simulink library "vmc"  (R2021b)
settings: Solver=VariableStepAuto  StartTime=0.0  StopTime=10.0  RelTol=1e-3
undefined symbols (not defined in the file or in its folder): AVMC_ACCDeltaTqIGain_X_kph, AVMC_ACCDeltaTqIGain_Y_mps2, AVMC_ACCDeltaTqIGainP2_X_kph, AVMC_ACCDeltaTqIGainP2_Y_mps2, AVMC_ACCDeltaTqPGain_X_kph, AVMC_ACCDeltaTqPGain_Y_kph, AVMC_ACCDeltaTqPGainP2_X_kph, AVMC_ACCDeltaTqPGainP2_Y_kph, AVMC_ACCLongSteadyCtrl_X_kph, AVMC_CCAccelCMD_X_kph, AVMC_CCAccelCMD_Y_kph, AVMC_CCDeltaTqIGain_X_kph, AVMC_CCDeltaTqIGain_Y_mps2, AVMC_CCDeltaTqPGain_X_kph, AVMC_CCDeltaTqPGain_Y_kph, AVMC_CCLongSteadyCtrl_X_kph, AVMC_DISCDeltaTqIGainP2_X_kph, AVMC_DISCDeltaTqIGainP2_Y_mps2, AVMC_ESCRegenOut_X_kph, AVMC_ESCRegenOut_Y_Deg, AVMC_ESCRegenOutEnSpd_X_Deg, AVMC_LatESCRegenOut_X_kph, AVMC_LatESCRegenOut_Y_Deg, AVMC_LongAccDeadZone_X_kph, AVMC_LongAccDeadZoneP2_X_kph, AVMC_LongAccFiltTs_X_Gps, AVMC_LongAccFiltTsP2_X_Gps, AVMC_MCPresBaseTq_X_bar, AVMC_MSAAccelCMD_X_kph, AVMC_MSAAccelCMD_Y_kph, AVMC_MSADeltaTqIGain_X_kph, AVMC_MSADeltaTqIGain_Y_mps2, AVMC_MSADeltaTqPGain_X_kph, AVMC_MSADeltaTqPGain_Y_kph, AVMC_MSALongSteadyCtrl_X_kph, AVMC_MSAPedalOvrd_X_kph, AVMC_MSASpdBand_X_kph, AVMC_OPDDisSlideRate_X_Deg, AVMC_RDCDetectTime_X_kph, AVMC_RDCDetectTime_Y_pct, AVMC_RDCEnSlideRate_X_Deg, AVMC_StESCYaw_X_kph, AVMC_StESCYaw_Y_Deg, AVMC_StESCYawCom_X_kph, AVMC_StESCYawCom_Y_Gps, AVMC_TMSpdBaseTq_X_rpm, C_TASK_10MS_S, C_TASK_5MS_S, DEG2RAD, Discrete, ENUM_ADASACCSTA_ACTIVE, ENUM_ADASACCSTA_OVERRIDE, ENUM_ADASACCSTA_STANDBY, ENUM_ADASMSASTA_ACTIVE, ENUM_ADASMSASTA_ERROR, ENUM_ADASMSASTA_OFF, ENUM_ADASMSASTA_OVERSPEED, ENUM_ADASMSASTA_STANDBY, ENUM_ADASMSASTA_UNDERSPEED, ENUM_ADASMSASTA_UNLIMIT ... (+254)
libraries: hcu_lib x57, simulink x49, ctrlSharedLib x6, simulink_extras x1
(part 1 of 9)
settings Model: Creator=FVT22120  LastModifiedBy=FVT23010

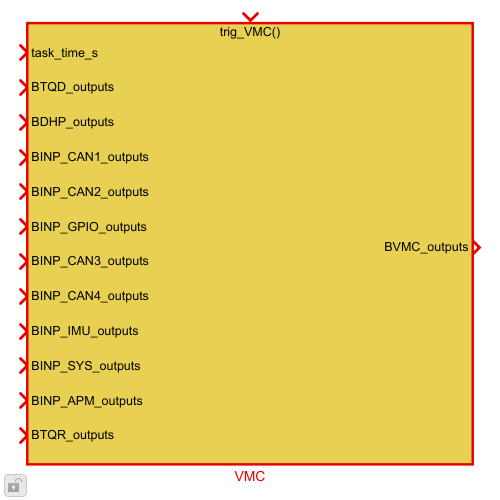
[thumbnail: Simulink's stored preview of the top-level diagram]
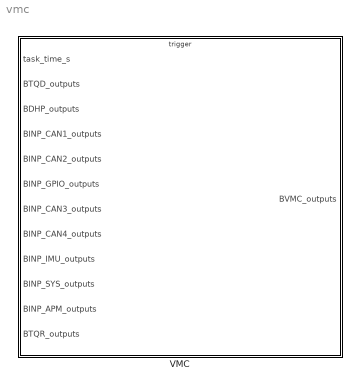
== system vmc ==
  VMC : Subsystem
      settings: RTWSystemCode=Nonreusable function  RTWFcnNameOpts=Use subsystem name  RTWFileNameOpts=Use subsystem name

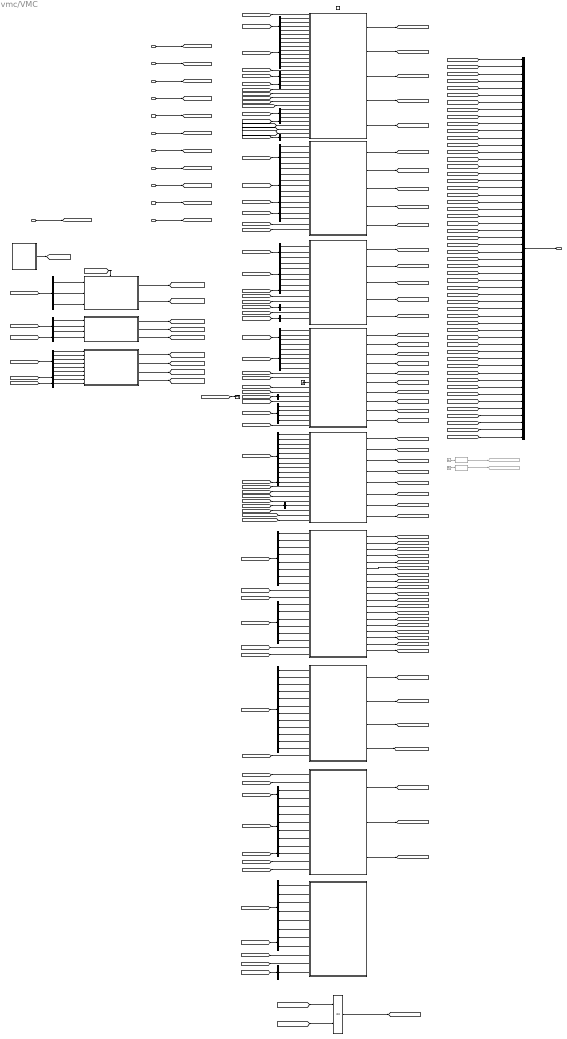
== system vmc/VMC ==
  note: Phase2_WAdd
  task_time_s : Inport
  BTQD_outputs : Inport  Port=2  OutDataTypeStr=Bus: BTQD_outputs
  BDHP_outputs : Inport  Port=3  OutDataTypeStr=Bus: BDHP_outputs
  BINP_CAN1_outputs : Inport  Port=4  OutDataTypeStr=Bus: BINP_CAN1_outputs
  BINP_CAN2_outputs : Inport  Port=5  OutDataTypeStr=Bus: BINP_CAN2_outputs  LockScale=on
  BINP_GPIO_outputs : Inport  Port=6  OutDataTypeStr=Bus: BINP_GPIO_outputs
  BINP_CAN3_outputs : Inport  Port=7  OutDataTypeStr=Bus: BINP_CAN3_outputs
  BINP_CAN4_outputs : Inport  Port=8  OutDataTypeStr=Bus: BINP_CAN4_outputs
  BINP_IMU_outputs : Inport  Port=9  OutDataTypeStr=Bus: BINP_IMU_outputs
  BINP_SYS_outputs : Inport  Port=10  OutDataTypeStr=Bus: BINP_SYS_outputs
  BINP_APM_outputs : Inport  Port=11  OutDataTypeStr=Bus: BINP_APM_outputs
  BTQR_outputs : Inport  Port=12  OutDataTypeStr=Bus: BTQR_outputs
  trig_VMC : TriggerPort  TriggerType=function-call  VariantControl=(inherit)  PortDimensions=1
  ACC_Function : Subsystem
  ACC_ReqAccelControl : Subsystem
  APS function : Subsystem
  Bus Creator : BusCreator  Inputs=54  OutDataTypeStr=Bus:BVMC_outputs  NonVirtualBus=on
  Bus Selector : BusSelector  OutputSignals=VINP_ACCRequiredAccel_mps2,VINP_ADASACCSta_enum,VINP_VehSpeed_kph,VINP_ACCSetSpeed_enum,VINP_ACCVehHoldReq_flg,VINP_MCPressure_bar,VINP_ESCADASSta_enum,VINP_TargetType_enum
  Bus Selector1 : BusSelector  OutputSignals=VTQD_ExternalTqAllow_flg,VTQD_DriverWhlTqDem_Nm,VTQD_LowIdleAccPedal_flg,VTQD_GearActualPosn_enum,VTQD_ExtDoorAllow_flg
  Bus Selector10 : BusSelector  OutputSignals=VINP_MemOffsetGyroX_raw16,VINP_MemOffsetGyroY_raw16,VINP_MemOffsetGyroZ_raw16,VINP_MemOffsetAccX_raw16,VINP_MemOffsetAccY_raw16,VINP_MemOffsetAccZ_raw16,VINP_SensingGyroX_raw16,VINP_SensingGyroY_raw16,VINP_SensingGyroZ_raw16,VINP_SensingAccX_raw16,VINP_SensingAccY_raw16,VINP_SensingAccZ_raw16
  Bus Selector11 : BusSelector  OutputSignals=VTQD_ExternalTqAllow_flg,VTQD_ExtShftAllow_flg,VTQD_ExtDoorAllow_flg,VTQD_GearActualPosn_enum
  Bus Selector12 : BusSelector  OutputSignals=VDHP_ActAPSPosn_pct
  Bus Selector13 : BusSelector  OutputSignals=VINP_GRADE_Deg,VINP_LatAccel_Gps,VINP_LongAccel_Gps,VINP_VehSpeed_kph,VINP_LFRawWhlSpeed_kph,VINP_RFRawWhlSpeed_kph,VINP_LRRawWhlSpeed_kph,VINP_RRRawWhlSpeed_kph,VINP_ACCSetSpeed_enum,VINP_TargetType_enum
  Bus Selector14 : BusSelector  OutputSignals=VINP_RegenMode_enum,VINP_SWCResUpSta_flg
  Bus Selector15 : BusSelector  OutputSignals=VINP_GPSLAT_s,VINP_GPSLONG_enum
  Bus Selector16 : BusSelector  OutputSignals=VINP_SetSpd_kph
  Bus Selector17 : BusSelector  OutputSignals=VINP_LFRawWhlSpeed_kph,VINP_RFRawWhlSpeed_kph,VINP_LRRawWhlSpeed_kph,VINP_RRRawWhlSpeed_kph,VINP_VehSpeed_kph,VINP_BrkPedalPos_pct,VINP_BrkSwSta_flg,VINP_LongAccel_Gps
  Bus Selector18 : BusSelector  OutputSignals=VTQD_AfterAvailableTqDemFr_Nm,VTQD_AfterAvailableTqDemRr_Nm,VTQD_EquivAccPedalSWSta_flg,VTQD_GearActualPosn_enum,VTQD_RegenMode_enum,VTQD_VehActSpd_kph
  Bus Selector19 : BusSelector  OutputSignals=VTQD_AfterAvailableTqDemFr_Nm,VTQD_AfterAvailableTqDemRr_Nm
  Bus Selector2 : BusSelector  OutputSignals=VTQD_DriverWhlTqDem_Nm,VTQD_ExternalTqAllow_flg,VTQD_LowIdleAccPedal_flg,VTQD_ExtDoorAllow_flg,VTQD_CreepBaseTqD_Nm
  Bus Selector20 : BusSelector  OutputSignals=VINP_ESCActive_flg,VINP_SASAngle_Deg,VINP_LatAccel_Gps,VINP_VehSpeed_kph,VINP_YawRate_degps,VINP_RDCActive_enum
  Bus Selector21 : BusSelector  OutputSignals=VINP_HoodSW_flg
  Bus Selector22 : BusSelector  OutputSignals=VINP_LFRawWhlSpeed_kph,VINP_RFRawWhlSpeed_kph,VINP_LRRawWhlSpeed_kph,VINP_RRRawWhlSpeed_kph,VINP_VehSpeed_kph,VINP_LongAccel_Gps
  Bus Selector23 : BusSelector  OutputSignals=VTQD_GearActualPosn_enum
  Bus Selector24 : BusSelector  OutputSignals=VINP_DIDGetDynoMode_flg
  Bus Selector25 : BusSelector  OutputSignals=VINP_DIDGetDynoMode_flg
  Bus Selector26 : BusSelector  OutputSignals=VINP_APSStaSystem_enum,VINP_APSVMCReqA_flg,VINP_APSShiftPosnReq_enum,VINP_APSSpeedCMD_kph,VINP_CAASVMCReqA_flg
  Bus Selector27 : BusSelector  OutputSignals=VINP_VehSpeed_kph
  Bus Selector28 : BusSelector  OutputSignals=VINP_VehSpeed_kph,VINP_ACCRequiredAccel_mps2,VINP_ADASACCSta_enum
  Bus Selector29 : BusSelector  OutputSignals=VINP_METERKPHCalcu_kph
  Bus Selector3 : BusSelector  OutputSignals=VINP_BrkSwSta_flg,VINP_VehSpeed_kph,VINP_BrkPedalPos_pct
  Bus Selector30 : BusSelector  OutputSignals=VINP_VehSpeed_kph,VINP_ACCRequiredAccel_mps2,VINP_ACCVehHoldReq_flg,VINP_ACCObjRelSpd_mps,VINP_ACCObjDist_m,VINP_TimeGapLevel_enum
  Bus Selector31 : BusSelector  OutputSignals=VTQD_FrEDUAvailBrkRgnTq_Nm,VTQD_RrEDUAvailBrkRgnTq_Nm
  Bus Selector32 : BusSelector  OutputSignals=VINP_VehSpeed_kph,VINP_LongAccel_Gps,VINP_GRADE_Deg
  Bus Selector33 : BusSelector  OutputSignals=VTQR_FrTMTqReq_Nm,VTQR_RrTMTqReq_Nm,VTQR_ACCHoldPdovrdInc_flg
  Bus Selector34 : BusSelector  OutputSignals=VINP_FrTMSpd_rpm,VINP_RrTMSpd_rpm
  Bus Selector35 : BusSelector  OutputSignals=VINP_METERKPHCalcu_kph
  Bus Selector36 : BusSelector  OutputSignals=VINP_METERKPHCalcu_kph
  Bus Selector37 : BusSelector  OutputSignals=VINP_ADASACCSta_enum,VINP_MCPressure_bar,VINP_BrkSwSta_flg,VINP_BrkPedalPos_pct
  Bus Selector4 : BusSelector  OutputSignals=VDHP_ActAPSPosn_pct
  Bus Selector5 : BusSelector  OutputSignals=VTQD_ExternalTqAllow_flg,VTQD_DriverWhlTqDem_Nm,VTQD_GearActualPosn_enum
  Bus Selector6 : BusSelector  OutputSignals=VINP_VehSpeed_kph
  Bus Selector7 : BusSelector  OutputSignals=VINP_ZoneSpdCtrlMode_enum,VINP_SetSpd_kph,VINP_SWCCANCELSta_flg,VINP_SWCResUpSta_flg,VINP_SWCSetdownSta_flg
  Bus Selector8 : BusSelector  OutputSignals=VINP_BrakeSWGPIO_flg
  Bus Selector9 : BusSelector  OutputSignals=VINP_ZoneSpdCtrlMode_enum,VINP_SetSpd_kph,VINP_SWCResUpSta_flg,VINP_SWCSetdownSta_flg,VINP_SWCCANCELSta_flg
  CruiseControlFunction : Subsystem
  Data Type Conversion : DataTypeConversion  Commented=on  OutDataTypeStr=boolean
  Data Type Conversion1 : DataTypeConversion  Commented=on  OutDataTypeStr=boolean
  Goto62 : Goto  Commented=on  GotoTag=VVMC_CAASCtrlAvail_flg
  Goto63 : Goto  Commented=on  GotoTag=VVMC_CAASActive_flg
  Ground5 : Ground
  Ground7 : Ground  Commented=on
  Ground8 : Ground  Commented=on
  IMU : Subsystem
  Logical Operator : Logic  Operator=OR  AllPortsSameDT=off  OutDataTypeStr=boolean
  Long Acceleration Calculation : Subsystem
  LongAccel_EstSlope : Subsystem  TreatAsAtomicUnit=on
  MSA function : Subsystem
  RDC Determination : Subsystem
  Scheduler : Stateflow chart  TreatAsAtomicUnit=on
  Slide Rate  Calculation : Subsystem
  Subsystem1 : Subsystem
  Terminator1 : Terminator
  Vehicle Speed Estimation : Subsystem
  BVMC_outputs : Outport  OutDataTypeStr=Bus:BVMC_outputs
  wires:
  Bus Creator/1 -> BVMC_outputs/1  "BVMC_outputs"
  [VVMC_MSAWhlTqReq_Nm] -> Bus Creator/9
  [VVMC_ACCCtrlAvail_flg] -> Bus Creator/1
  [VVMC_CCPedalOvrd_flg] -> Bus Creator/16
  [VVMC_ADASWhlTqReq_Nm] -> Bus Creator/3
  [VVMC_ACCPedalOvrd_flg] -> Bus Creator/2
  [VVMC_MSAActive_flg] -> Bus Creator/11
  [VVMC_APSSpeedCMD_kph] -> Bus Creator/14
  [VVMC_MSACtrlSta_enum] -> Bus Creator/7
  [VVMC_APSCtrlAvail_flg] -> Bus Creator/12
  [VVMC_CruzActive_flg] -> Bus Creator/10
  [VVMC_APSActive_flg] -> Bus Creator/13
  [VVMC_ADASActive_flg] -> Bus Creator/4
  [VVMC_CCCtrlSta_enum] -> Bus Creator/5
  [VVMC_APSShiftPosnReq_enum] -> Bus Creator/15
  [VVMC_CruzWhlTqReq_Nm] -> Bus Creator/8
  [VVMC_CCMSASpdWar_flg] -> Bus Creator/6
  MSA function/4(VVMC_MSAActive_flg) -> [VVMC_MSAActive_flg]
  MSA function/3(VVMC_MSASpdWar_flg) -> [VVMC_MSASpdWar_flg]
  MSA function/2(VVMC_MSAWhlTqReq_Nm) -> [VVMC_MSAWhlTqReq_Nm]
  MSA function/1(VVMC_MSACtrlSta_enum) -> [VVMC_MSACtrlSta_enum]
  [VVMC_LongAcc_Gps] -> MSA function/10(VVMC_LongAcc_Gps)
  [BINP_CAN1_outputs] -> Bus Selector6/1
  Bus Selector7/2 -> MSA function/5(VINP_SetSpd_kph)  "<VINP_SetSpd_kph>"
  Bus Selector7/1 -> MSA function/4(VINP_ZoneSpdCrlMode_enum)  "<VINP_ZoneSpdCtrlMode_enum>"
  Bus Selector5/2 -> MSA function/2(VTQD_DriverWhlTqDem_Nm)  "<VTQD_DriverWhlTqDem_Nm>"
  Bus Selector5/1 -> MSA function/1(VTQD_ExternalTqAllow_flg)  "<VTQD_ExternalTqAllow_flg>"
  CruiseControlFunction/1(VVMC_CCCtrlSta_enum) -> [VVMC_CCCtrlSta_enum]
  CruiseControlFunction/3(VVMC_CruzWhlTqReq_N m) -> [VVMC_CruzWhlTqReq_Nm]
  CruiseControlFunction/5(VVMC_CCPedalOvrd_flg) -> [VVMC_CCPedalOvrd_flg]
  CruiseControlFunction/2(VVMC_CCSpdWar_flg) -> [VVMC_CCSpdWar_flg]
  CruiseControlFunction/4(VVMC_CruzActive_flg) -> [VVMC_CruzActive_flg]
  [VVMC_LongAcc_Gps] -> CruiseControlFunction/15(VVMC_LongAcc_Gps)
  Bus Selector3/2 -> CruiseControlFunction/13(VINP_VehSpeed_kph)  "<VINP_VehSpeed_kph>"
  Bus Selector3/1 -> CruiseControlFunction/12(VINP_BrkSwSta_flg)  "<VINP_BrkSwSta_flg>"
  Bus Selector8/1 -> CruiseControlFunction/11(VINP_BrakeSWGPIO_flg)  "<VINP_BrakeSWGPIO_flg>"
  Bus Selector9/5 -> CruiseControlFunction/10(VINP_SWCCANCELSta_flg)  "<VINP_SWCCANCELSta_flg>"
  Bus Selector9/4 -> CruiseControlFunction/9(VINP_SWCSetdownSta_flg)  "<VINP_SWCSetdownSta_flg>"
  Bus Selector9/3 -> CruiseControlFunction/8(VINP_SWCResUpSta_flg)  "<VINP_SWCResUpSta_flg>"
  Bus Selector9/2 -> CruiseControlFunction/7(VINP_SetSpd_kph)  "<VINP_SetSpd_kph>"
  Bus Selector9/1 -> CruiseControlFunction/6(VINP_ZoneSpdCrlMode_enum)  "<VINP_ZoneSpdCtrlMode_enum>"
  Bus Selector1/3 -> CruiseControlFunction/3(VTQD_LowIdleAccPedal_flg)  "<VTQD_LowIdleAccPedal_flg>"
  Bus Selector1/2 -> CruiseControlFunction/2(VTQD_DriverWhlTqDem_Nm)  "<VTQD_DriverWhlTqDem_Nm>"
  Bus Selector1/1 -> CruiseControlFunction/1(VTQD_ExternalTqAllow_flg)  "<VTQD_ExternalTqAllow_flg>"
  BINP_CAN2_outputs/1 -> [BINP_CAN2_outputs]
  task_time_s/1 -> [task_time_s]  "task_time_s"
  BTQD_outputs/1 -> [BTQD_outputs]
  [BTQD_outputs] -> Bus Selector1/1
  [BINP_CAN1_outputs] -> Bus Selector3/1
  [VVMC_CCSpdWar_flg] -> Logical Operator/1
  [VVMC_MSASpdWar_flg] -> Logical Operator/2
  Logical Operator/1 -> [VVMC_CCMSASpdWar_flg]  "VVMC_CCMSASpdWar_flg"
  [BTQD_outputs] -> Bus Selector5/1
  BINP_GPIO_outputs/1 -> [BINP_GPIO_outputs]
  [BINP_GPIO_outputs] -> Bus Selector8/1
  BINP_CAN3_outputs/1 -> [BINP_CAN3_outputs]
  [BINP_CAN4_outputs] -> Bus Selector7/1
  [BINP_CAN4_outputs] -> Bus Selector9/1
  BDHP_outputs/1 -> [BDHP_outputs]
  BINP_CAN1_outputs/1 -> [BINP_CAN1_outputs]
  [BTQD_outputs] -> Bus Selector11/1
  APS function/1(VVMC_APSCtrlAvail_flg) -> [VVMC_APSCtrlAvail_flg]
  APS function/4(VVMC_APSShiftPosnReq_enum) -> [VVMC_APSShiftPosnReq_enum]
  Long Acceleration Calculation/1(VVMC_LongAcc_Gps) -> [VVMC_LongAcc_Gps]
  APS function/3(VVMC_APSSpeedCMD_kph) -> [VVMC_APSSpeedCMD_kph]
  Bus Selector11/1 -> APS function/1(VTQD_ExternalTqAllow_flg)  "<VTQD_ExternalTqAllow_flg>"
  [task_time_s] -> APS function/10(task_time_s)  "task_time_s"
  APS function/2(VVMC_APSActive_flg) -> [VVMC_APSActive_flg]
  BINP_CAN4_outputs/1 -> [BINP_CAN4_outputs]
  [VVMC_LongAcc_Gps] -> Bus Creator/17
  [task_time_s] -> Long Acceleration Calculation/14(task_time_s)  "task_time_s"
  Bus Selector1/4 -> CruiseControlFunction/4(VTQD_GearActualPosn_enum)  "<VTQD_GearActualPosn_enum>"
  Bus Selector11/2 -> APS function/2(VTQD_ExtShiftAllow_flg)  "<VTQD_ExtShftAllow_flg>"
  [VVMC_ADASNegReq_flg] -> Bus Creator/18
  Bus Selector3/3 -> CruiseControlFunction/14(VINP_BrkPedalPos_pct)  "<VINP_BrkPedalPos_pct>"
  Bus Selector17/6 -> Slide Rate  Calculation/6(VINP_BrkPedalPos_pct)  "<VINP_BrkPedalPos_pct>"
  Bus Selector17/7 -> Slide Rate  Calculation/7(VINP_BrkSwSta_flg)  "<VINP_BrkSwSta_flg>"
  Bus Selector17/4 -> Slide Rate  Calculation/4(VINP_RRRawWhlSpeed_kph)  "<VINP_RRRawWhlSpeed_kph>"
  Slide Rate  Calculation/4(VVMC_LRWhlSpdSlideRate_pct) -> [VVMC_LRWhlSpdSlideRate_pct]
  Slide Rate  Calculation/14(VVMC_ActRFSlideRate_pct) -> [VVMC_ActRFSlideRate_pct]
  Slide Rate  Calculation/8(VVMC_LR4WhlSpdSlideRate_pct) -> [VVMC_LR4WhlSpdSlideRate_pct]
  Slide Rate  Calculation/15(VVMC_ActLRSlideRate_pct) -> [VVMC_ActLRSlideRate_pct]
  Slide Rate  Calculation/16(VVMC_ActRRSlideRate_pct) -> [VVMC_ActRRSlideRate_pct]
  Slide Rate  Calculation/1(VVMC_RawWhlSpdSlideRate_pct) -> [VVMC_RawWhlSpdSlideRate_pct]
  Slide Rate  Calculation/12(VVMC_ActMaxSlideRate_pct) -> [VVMC_ActMaxSlideRate_pct]
  Slide Rate  Calculation/3(VVMC_RFWhlSpdSlideRate_pct) -> [VVMC_RFWhlSpdSlideRate_pct]
  Slide Rate  Calculation/2(VVMC_LFWhlSpdSlideRate_pct) -> [VVMC_LFWhlSpdSlideRate_pct]
  Slide Rate  Calculation/9(VVMC_RR4WhlSpdSlideRate_pct) -> [VVMC_RR4WhlSpdSlideRate_pct]
  Slide Rate  Calculation/5(VVMC_RRWhlSpdSlideRate_pct) -> [VVMC_RRWhlSpdSlideRate_pct]
  Bus Selector18/3 -> Slide Rate  Calculation/13(VTQD_EquivAccPedalSWSta_flg)  "<VTQD_EquivAccPedalSWSta_flg>"
  Bus Selector18/1 -> Slide Rate  Calculation/11(VTQD_AfterAvailableTqDemFr_Nm)  "<VTQD_AfterAvailableTqDemFr_Nm>"
  Bus Selector17/2 -> Slide Rate  Calculation/2(VINP_RFRawWhlSpeed_kph)  "<VINP_RFRawWhlSpeed_kph>"
  Bus Selector17/5 -> Slide Rate  Calculation/5(VINP_VehSpeed_kph)  "<VINP_VehSpeed_kph>"
  Bus Selector17/3 -> Slide Rate  Calculation/3(VINP_LRRawWhlSpeed_kph)  "<VINP_LRRawWhlSpeed_kph>"
  [task_time_s] -> Slide Rate  Calculation/10(task_time_s)  "task_time_s"
  [BTQD_outputs] -> Bus Selector18/1
  [BINP_CAN1_outputs] -> Bus Selector17/1
  Slide Rate  Calculation/10(VVMC_PredictVehSpd_kph) -> [VVMC_PredictVehSpd_kph]
  [VVMC_LongAcc_Gps] -> Slide Rate  Calculation/9(VVMC_LongAcc_Gps)
  Slide Rate  Calculation/18(VVMC_AltRWhlSlideRate_pct) -> [VVMC_AltRWhlSlideRate_pct]
  Slide Rate  Calculation/17(VVMC_AltLWhlSlideRate_pct) -> [VVMC_AltLWhlSlideRate_pct]
  Bus Selector17/1 -> Slide Rate  Calculation/1(VINP_LFRawWhlSpeed_kph)  "<VINP_LFRawWhlSpeed_kph>"
  Slide Rate  Calculation/6(VVMC_LF4WhlSpdSlideRate_pct) -> [VVMC_LF4WhlSpdSlideRate_pct]
  Slide Rate  Calculation/7(VVMC_RF4WhlSpdSlideRate_pct) -> [VVMC_RF4WhlSpdSlideRate_pct]
  Slide Rate  Calculation/19(VVMC_AltWhlSlideRate_pct) -> [VVMC_AltWhlSlideRate_pct]
  Slide Rate  Calculation/13(VVMC_ActLFSlideRate_pct) -> [VVMC_ActLFSlideRate_pct]
  Bus Selector18/2 -> Slide Rate  Calculation/12(VTQD_AfterAvailableTqDemRr_Nm)  "<VTQD_AfterAvailableTqDemRr_Nm>"
  [VVMC_ADASActive_flg] -> Long Acceleration Calculation/12(VVMC_ADASActive_flg)
  Bus Selector16/1 -> Long Acceleration Calculation/11(VINP_SetSpd_kph)  "<VINP_SetSpd_kph>"
  Bus Selector13/9 -> Long Acceleration Calculation/9(VINP_ACCSetSpeed_enum)  "<VINP_ACCSetSpeed_enum>"
  Bus Selector13/7 -> Long Acceleration Calculation/7(VINP_LRRawWhlSpeed_kph)  "<VINP_LRRawWhlSpeed_kph>"
  Bus Selector13/6 -> Long Acceleration Calculation/6(VINP_RFRawWhlSpeed_kph)  "<VINP_RFRawWhlSpeed_kph>"
  Bus Selector13/5 -> Long Acceleration Calculation/5(VINP_LFRawWhlSpeed_kph)  "<VINP_LFRawWhlSpeed_kph>"
  Bus Selector13/4 -> Long Acceleration Calculation/4(VINP_VehSpeed_kph)  "<VINP_VehSpeed_kph>"
  Bus Selector13/3 -> Long Acceleration Calculation/3(VINP_LongAccel_Gps)  "<VINP_LongAccel_Gps>"
  [VVMC_CruzActive_flg] -> Long Acceleration Calculation/13(VVMC_CruzActive_flg)
  [BINP_CAN4_outputs] -> Bus Selector16/1
  Bus Selector13/2 -> Long Acceleration Calculation/2(VINP_LatAccel_Gps)  "<VINP_LatAccel_Gps>"
  Bus Selector13/1 -> Long Acceleration Calculation/1(VINP_GRADE_deg)  "<VINP_GRADE_Deg>"
  Bus Selector13/8 -> Long Acceleration Calculation/8(VINP_RRRawWhlSpeed_kph)  "<VINP_RRRawWhlSpeed_kph>"
  [BINP_CAN1_outputs] -> Bus Selector13/1
  Bus Selector13/10 -> Long Acceleration Calculation/10(VINP_TargetType_enum)  "<VINP_TargetType_enum>"
  Long Acceleration Calculation/2(VVMC_LFWhlSpeedRollAve_kph) -> [VVMC_LFWhlSpeedRollAve_kph]
  Long Acceleration Calculation/3(VVMC_RFWhlSpeedRollAve_kph) -> [VVMC_RFWhlSpeedRollAve_kph]
  Long Acceleration Calculation/4(VVMC_LRWhlSpeedRollAve_kph) -> [VVMC_LRWhlSpeedRollAve_kph]
  Long Acceleration Calculation/5(VVMC_RRWhlSpeedRollAve_kph) -> [VVMC_RRWhlSpeedRollAve_kph]
  Long Acceleration Calculation/6(VVMC_CalMeterSpeed_kph) -> [VVMC_CalMeterSpeed_kph]
  [BTQD_outputs] -> APS function/11(BTQD_outputs)  "BTQD_outputs"
  [VVMC_ADASActive_flg] -> APS function/13(VVMC_ADASActive_flg)
  APS function/5(VVMC_APSStaSys_enum) -> [VVMC_APSStaSys_enum]
  APS function/6(VVMC_APSDecReqA_flg) -> [VVMC_APSDecReqA_flg]
  APS function/7(VVMC_APSDecReq_mps2) -> [VVMC_APSDecReq_mps2]
  APS function/8(VVMC_APSReq_enum) -> [VVMC_APSReq_enum]
  Bus Selector5/3 -> MSA function/3(VTQD_GearActualPosn_enum)  "<VTQD_GearActualPosn_enum>"
  Bus Selector7/3 -> MSA function/6(VINP_SWCCANCELSta_flg)  "<VINP_SWCCANCELSta_flg>"
  Bus Selector6/1 -> MSA function/9(VINP_VehSpeed_kph)  "<VINP_VehSpeed_kph>"
  [BDHP_outputs] -> Bus Selector12/1
  [task_time_s] -> MSA function/11(task_time_s)  "task_time_s"
  Bus Selector12/1 -> MSA function/12(VDHP_ActAPSPosn_pct)  "<VDHP_ActAPSPosn_pct>"
  [VVMC_CalMeterSpeed_kph] -> MSA function/13(VVMC_CalMeterSpeed_kph)
  [VVMC_CalMeterSpeed_kph] -> CruiseControlFunction/16(VVMC_CalMeterSpeed_kph)
  [VVMC_APSStaSys_enum] -> Bus Creator/19
  [VVMC_APSDecReqA_flg] -> Bus Creator/20
  [VVMC_APSDecReq_mps2] -> Bus Creator/21
  [VVMC_APSReq_enum] -> Bus Creator/22
  [VVMC_LFWhlSpeedRollAve_kph] -> Bus Creator/23
  [VVMC_RFWhlSpeedRollAve_kph] -> Bus Creator/24
  [VVMC_LRWhlSpeedRollAve_kph] -> Bus Creator/25
  [VVMC_RRWhlSpeedRollAve_kph] -> Bus Creator/26
  [VVMC_RawWhlSpdSlideRate_pct] -> Bus Creator/27
  [VVMC_LFWhlSpdSlideRate_pct] -> Bus Creator/28
  [VVMC_RFWhlSpdSlideRate_pct] -> Bus Creator/29
  [VVMC_LRWhlSpdSlideRate_pct] -> Bus Creator/30
  [VVMC_RRWhlSpdSlideRate_pct] -> Bus Creator/31
  [VVMC_PredictVehSpd_kph] -> Bus Creator/32
  [VVMC_4WhlSpdSlideRate_pct] -> Bus Creator/33
  [VVMC_LF4WhlSpdSlideRate_pct] -> Bus Creator/34
  [VVMC_RF4WhlSpdSlideRate_pct] -> Bus Creator/35
  [VVMC_LR4WhlSpdSlideRate_pct] -> Bus Creator/36
  [VVMC_RR4WhlSpdSlideRate_pct] -> Bus Creator/37
  [VVMC_ActMaxSlideRate_pct] -> Bus Creator/38
  [VVMC_ActLFSlideRate_pct] -> Bus Creator/39
  [VVMC_ActRFSlideRate_pct] -> Bus Creator/40
  [VVMC_ActLRSlideRate_pct] -> Bus Creator/41
  [VVMC_ActRRSlideRate_pct] -> Bus Creator/42
  [VVMC_AltLWhlSlideRate_pct] -> Bus Creator/43
  [VVMC_AltRWhlSlideRate_pct] -> Bus Creator/44
  [VVMC_AltWhlSlideRate_pct] -> Bus Creator/45
  Bus Selector7/4 -> MSA function/7(VINP_SWCResUpSta_flg)  "<VINP_SWCResUpSta_flg>"
  Bus Selector7/5 -> MSA function/8(VINP_SWCSetdownSta_flg)  "<VINP_SWCSetdownSta_flg>"
  [VVMC_MSAActive_flg] -> Long Acceleration Calculation/15(VVMC_MSAActive_flg)
  Long Acceleration Calculation/7(VVMC_EstSlope_Deg) -> [VVMC_EstSlope_Deg]
  [VVMC_EstSlope_Deg] -> Bus Creator/46
  Slide Rate  Calculation/11(VVMC_4WhlSpdSlideRate_pct) -> [VVMC_4WhlSpdSlideRate_pct]
  Bus Selector21/1 -> MSA function/14(VINP_HoodSW_flg)  "<VINP_HoodSW_flg>"
  [BINP_GPIO_outputs] -> Bus Selector21/1
  [VVMC_RWDRDCActive_enum] -> Bus Creator/47
  Bus Selector1/5 -> CruiseControlFunction/5(VTQD_ExtDoorAllow_flg)  "<VTQD_ExtDoorAllow_flg>"
  Bus Selector11/3 -> APS function/3(VTQD_ExtDoorAllow_flg)  "<VTQD_ExtDoorAllow_flg>"
  BINP_IMU_outputs/1 -> [BINP_IMU_outputs]
  [BINP_IMU_outputs] -> Bus Selector10/1
  Bus Selector10/1 -> IMU/1(VINP_MemOffsetGyroX_raw16)  "<VINP_MemOffsetGyroX_raw16>"
  Bus Selector10/2 -> IMU/2(VINP_MemOffsetGyroY_raw16)  "<VINP_MemOffsetGyroY_raw16>"
  Bus Selector10/3 -> IMU/3(VINP_MemOffsetGyroZ_raw16)  "<VINP_MemOffsetGyroZ_raw16>"
  Bus Selector10/4 -> IMU/4(VINP_MemOffsetAccX_raw16)  "<VINP_MemOffsetAccX_raw16>"
  Bus Selector10/5 -> IMU/5(VINP_MemOffsetAccY_raw16)  "<VINP_MemOffsetAccY_raw16>"
  Bus Selector10/6 -> IMU/6(VINP_MemOffsetAccZ_raw16)  "<VINP_MemOffsetAccZ_raw16>"
  Bus Selector10/7 -> IMU/7(VINP_SensingGyroX_raw16)  "<VINP_SensingGyroX_raw16>"
  Bus Selector10/8 -> IMU/8(VINP_SensingGyroY_raw16)  "<VINP_SensingGyroY_raw16>"
  Bus Selector10/9 -> IMU/9(VINP_SensingGyroZ_raw16)  "<VINP_SensingGyroZ_raw16>"
  Bus Selector10/10 -> IMU/10(VINP_SensingAccX_raw16)  "<VINP_SensingAccX_raw16>"
  Bus Selector10/11 -> IMU/11(VINP_SensingAccY_raw16)  "<VINP_SensingAccY_raw16>"
  Bus Selector10/12 -> IMU/12(VINP_SensingAccZ_raw16)  "<VINP_SensingAccZ_raw16>"
  IMU/1(VVMC_IMUEnaCmd_flg) -> [VVMC_IMUEnaCmd_flg]
  [VVMC_IMUEnaCmd_flg] -> Bus Creator/48
  Bus Selector18/4 -> Slide Rate  Calculation/14(VTQD_GearActualPosn_enum)  "<VTQD_GearActualPosn_enum>"
  [BINP_CAN1_outputs] -> Bus Selector20/1
  Bus Selector20/4 -> RDC Determination/8(VINP_VehSpeed_kph)  "<VINP_VehSpeed_kph>"
  [VVMC_ActMaxSlideRate_pct] -> RDC Determination/2(VVMC_ActMaxSlideRate_pct)
  Bus Selector20/2 -> RDC Determination/6(VINP_SASAngle_Deg)  "<VINP_SASAngle_Deg>"
  Bus Selector19/1 -> RDC Determination/3(VTQD_AfterAvailableTqDemFr_Nm)  "<VTQD_AfterAvailableTqDemFr_Nm>"
  RDC Determination/1(VVMC_RWDRDCActive_enum) -> [VVMC_RWDRDCActive_enum]
  Bus Selector20/3 -> RDC Determination/7(VINP_LatAccel_Gps)  "<VINP_LatAccel_Gps>"
  [BTQD_outputs] -> Bus Selector19/1
  Bus Selector20/6 -> RDC Determination/10(VINP_RDCActive_enum)  "<VINP_RDCActive_enum>"
  Bus Selector20/5 -> RDC Determination/9(VINP_YawRate_degps)  "<VINP_YawRate_degps>"
  [task_time_s] -> RDC Determination/1(task_time_s)  "task_time_s"
  Bus Selector19/2 -> RDC Determination/4(VTQD_AfterAvailableTqDemRr_Nm)  "<VTQD_AfterAvailableTqDemRr_Nm>"
  Bus Selector20/1 -> RDC Determination/5(VINP_ESCActive_flg)  "<VINP_ESCActive_flg>"
  RDC Determination/3(VVMC_ActStESCYaw_degps) -> [VVMC_ActStESCYaw_Dps]
  RDC Determination/2(VVMC_RDCEnSlideRate_pct) -> [VVMC_RDCEnSlideRate_pct]
  [BINP_CAN4_outputs] -> Terminator1/1
  [BINP_APM_outputs] -> APS function/14(BINP_APM_outputs)  "BINP_APM_outputs"
  Bus Selector11/4 -> APS function/4(VTQD_GearActualPosn_enum)  "<VTQD_GearActualPosn_enum>"
  [VVMC_RDCEnSlideRate_pct] -> Bus Creator/49
  Bus Selector17/8 -> Slide Rate  Calculation/8(VINP_LongAccel_Gps)  "<VINP_LongAccel_Gps>"
  [task_time_s] -> Vehicle Speed Estimation/10(task_time_s)  "task_time_s"
  [VVMC_LongAcc_Gps] -> Vehicle Speed Estimation/9(VVMC_LongAcc_Gps)
  Bus Selector22/4 -> Vehicle Speed Estimation/4(VINP_RRRawWhlSpeed_kph)  "<VINP_RRRawWhlSpeed_kph>"
  Bus Selector22/5 -> Vehicle Speed Estimation/5(VINP_VehSpeed_kph)  "<VINP_VehSpeed_kph>"
  Bus Selector22/6 -> Vehicle Speed Estimation/6(VINP_LongAccel_Gps)  "<VINP_LongAccel_Gps>"
  [BTQD_outputs] -> Bus Selector23/1
  Bus Selector22/3 -> Vehicle Speed Estimation/3(VINP_LRRawWhlSpeed_kph)  "<VINP_LRRawWhlSpeed_kph>"
  Bus Selector22/2 -> Vehicle Speed Estimation/2(VINP_RFRawWhlSpeed_kph)  "<VINP_RFRawWhlSpeed_kph>"
  Bus Selector22/1 -> Vehicle Speed Estimation/1(VINP_LFRawWhlSpeed_kph)  "<VINP_LFRawWhlSpeed_kph>"
  Bus Selector23/1 -> Vehicle Speed Estimation/11(VTQD_GearActualPosn_enum)  "<VTQD_GearActualPosn_enum>"
  [BINP_CAN1_outputs] -> Bus Selector22/1
  Ground5/1 -> APS function/12(VINP_SCPSystemMode_enum)
  [VVMC_ActStESCYaw_Dps] -> Bus Creator/50
  [VVMC_CAASCtrlAvail_flg] -> Bus Creator/51
  [VVMC_CAASActive_flg] -> Bus Creator/52
  Ground7/1 -> Data Type Conversion/1
  Data Type Conversion/1 -> Goto62/1  "VVMC_CAASCtrlAvail_flg"
  Data Type Conversion1/1 -> Goto63/1  "VVMC_CAASActive_flg"
  Ground8/1 -> Data Type Conversion1/1
  [BINP_CAN2_outputs] -> Bus Selector15/1
  Bus Selector15/1 -> Vehicle Speed Estimation/7(VINP_GPSLAT_sec)  "<VINP_GPSLAT_s>"
  Bus Selector15/2 -> Vehicle Speed Estimation/8(VINP_GPSLONG_sec)  "<VINP_GPSLONG_enum>"
  BINP_SYS_outputs/1 -> [BINP_SYS_outputs]
  [BINP_SYS_outputs] -> Bus Selector24/1
  Bus Selector24/1 -> RDC Determination/11(VINP_DIDGetDynoMode_flg)  "<VINP_DIDGetDynoMode_flg>"
  Bus Selector25/1 -> Long Acceleration Calculation/16(VINP_DIDGetDynoMode_flg)  "<VINP_DIDGetDynoMode_flg>"
  [BINP_SYS_outputs] -> Bus Selector25/1
  [BINP_APM_outputs] -> Bus Selector26/1
  Bus Selector26/1 -> APS function/5(VINP_APSStaSys_enum)  "<VINP_APSStaSystem_enum>"
  Bus Selector26/2 -> APS function/6(VINP_APSVMCReqA_flg)  "<VINP_APSVMCReqA_flg>"
  Bus Selector26/3 -> APS function/7(VINP_APSShiftPosnReq_enum)  "<VINP_APSShiftPosnReq_enum>"
  Bus Selector26/4 -> APS function/8(VINP_APSSpeedCMD_kph)  "<VINP_APSSpeedCMD_kph>"
  Bus Selector26/5 -> APS function/9(VINP_CAASVMCReqA_flg)  "<VINP_CAASVMCReqA_flg>"
  BINP_APM_outputs/1 -> [BINP_APM_outputs]
  APS function/10(VVMC_CAASActive_flg) -> [VVMC_CAASActive_flg]
  APS function/9(VVMC_CAASCtrlAvail_flg) -> [VVMC_CAASCtrlAvail_flg]
  Bus Selector27/1 -> APS function/15(VINP_VehSpeed_kph)  "<VINP_VehSpeed_kph>"
  [BINP_CAN1_outputs] -> Bus Selector27/1
  [VVMC_CruzActive_flg] -> APS function/16(VVMC_CruzActive_flg)
  IMU/2(VVMC_CalibratedAccX_G) -> [VVMC_CalibratedAccX_G]
  [VVMC_CalibratedAccX_G] -> Long Acceleration Calculation/17(VVMC_CalibratedAccX_G)
  [VVMC_CalibratedAccX_G] -> Slide Rate  Calculation/17(VVMC_CalibratedAccX_G)
  IMU/3(VVMC_CalibratedGyroY_Dps) -> [VVMC_CalibratedGyroY_Dps]
  IMU/4(VVMC_CalibratedAccY_G) -> [VVMC_CalibratedAccY_G]
  [VVMC_CalibratedGyroY_Dps] -> RDC Determination/12(VVMC_CalibratedGyroY_Dps)
  [VVMC_CalibratedAccY_G] -> RDC Determination/13(VVMC_CalibratedAccY_G)
  [VVMC_CalibratedGyroY_Dps] -> Bus Creator/53
  [VVMC_EstSlope_Deg] -> Slide Rate  Calculation/18(VVMC_EstSlope_Deg)
  Bus Selector18/5 -> Slide Rate  Calculation/15(VTQD_RegenMode_enum)  "<VTQD_RegenMode_enum>"
  Bus Selector18/6 -> Slide Rate  Calculation/16(VTQD_VehActSpd_kph)  "<VTQD_VehActSpd_kph>"
  [task_time_s] -> IMU/13(task_time_s)  "task_time_s"
  LongAccel_EstSlope/1(VVMC_EstSlope_Deg) -> [VVMC_EstSlopeCal_Deg]
  ACC_ReqAccelControl/3(VVMC_ACCSpdCtrl_flg) -> [VVMC_ACCSpdCtrl_flg]
  Bus Selector36/1 -> Subsystem1/9(VINP_METERKPHCalcu_kph)  "<VINP_METERKPHCalcu_kph>"
  Bus Selector30/5 -> Subsystem1/5(VINP_ACCObjDist_m)  "<VINP_ACCObjDist_m>"
  [BINP_CAN2_outputs] -> Bus Selector36/1
  Bus Selector30/6 -> Subsystem1/6(VINP_TimeGapLevel_enum)  "<VINP_TimeGapLevel_enum>"
  [BTQD_outputs] -> Bus Selector31/1
  Bus Selector31/1 -> Subsystem1/7(VTQD_FrEDUAvailBrkRgnTq_Nm)  "<VTQD_FrEDUAvailBrkRgnTq_Nm>"
  Bus Selector30/1 -> Subsystem1/1(VINP_VehSpeed_kph)  "<VINP_VehSpeed_kph>"
  [BINP_CAN1_outputs] -> Bus Selector32/1
  Subsystem1/1(VVMC_AccelTurnHold_flg) -> [VVMC_AccelTurnHold_flg]
  Subsystem1/3(VVMC_TimeGapJudge_flag) -> [VVMC_TimeGapJudge_flag]
  Bus Selector32/1 -> LongAccel_EstSlope/1(VINP_VehSpeed_kph)  "<VINP_VehSpeed_kph>"
  Bus Selector28/1 -> ACC_ReqAccelControl/1(VINP_VehSpeed_kph)  "<VINP_VehSpeed_kph>"
  [BINP_CAN2_outputs] -> Bus Selector29/1
  Scheduler/1(Trigger_10ms_1()) -> [Trigger_10ms_1]
  LongAccel_EstSlope/2(VVMC_LongAccelCalcuByVehSpd_gps) -> [VVMC_LongAccelCalcuByVehSpd_gps]
  [BINP_CAN1_outputs] -> Bus Selector30/1
  Bus Selector29/1 -> ACC_ReqAccelControl/4(VVMC_MeterIndSpeedForCalcu_kph)  "<VINP_METERKPHCalcu_kph>"
  Bus Selector31/2 -> Subsystem1/8(VTQD_RrEDUAvailBrkRgnTq_Nm)  "<VTQD_RrEDUAvailBrkRgnTq_Nm>"
  ACC_ReqAccelControl/1(VVMC_AfterCtrlACCReqAccel_mps2) -> [VVMC_AfterCtrlACCReqAccel_mps2]
  Bus Selector32/3 -> LongAccel_EstSlope/3(VINP_GRADE_deg)  "<VINP_GRADE_Deg>"
  [BINP_CAN1_outputs] -> Bus Selector28/1
  Bus Selector28/2 -> ACC_ReqAccelControl/2(VINP_ACCRequiredAccel_mps2)  "<VINP_ACCRequiredAccel_mps2>"
  Subsystem1/4(VVMC_AllowSetSpd_flg) -> [VVMC_AllowSetSpd_flg]
  [Trigger_10ms_1] -> LongAccel_EstSlope/Trigger
  Bus Selector30/3 -> Subsystem1/3(VINP_ACCVehHoldReq_flg)  "<VINP_ACCVehHoldReq_flg>"
  Subsystem1/2(VVMC_TotalAvailBrkRgnTq_Nm) -> [VVMC_TotalAvailBrkRgnTq_Nm]
  Bus Selector28/3 -> ACC_ReqAccelControl/3(VINP_ADASACCSta_enum)  "<VINP_ADASACCSta_enum>"
  Bus Selector32/2 -> LongAccel_EstSlope/2(VINP_LongAccel_Gps)  "<VINP_LongAccel_Gps>"
  ACC_ReqAccelControl/2(VVMC_ACCReqSpdMemory_kph) -> [VVMC_ACCReqSpdMemory_kph]
  Bus Selector30/4 -> Subsystem1/4(VINP_ACCObjRelSpd_mps)  "<VINP_ACCObjRelSpd_mps>"
  Bus Selector30/2 -> Subsystem1/2(VINP_ACCRequiredAccel_mps2)  "<VINP_ACCRequiredAccel_mps2>"
  BTQR_outputs/1 -> [BTQR_outputs]
  Bus Selector2/5 -> ACC_Function/6(VTQD_CreepBaseTqD_Nm)  "<VTQD_CreepBaseTqD_Nm>"
  Bus Selector34/1 -> ACC_Function/16(VINP_FrTMSpd_rpm)  "<VINP_FrTMSpd_rpm>"
  Bus Selector/2 -> ACC_Function/8(VINP_ADASACCSta_enum)  "<VINP_ADASACCSta_enum>"
  Bus Selector14/2 -> ACC_Function/19(VINP_SWCResUpSta_flg)  "<VINP_SWCResUpSta_flg>"
  Bus Selector33/3 -> ACC_Function/27(VTQR_ACCHoldPdovrdInc_flg)  "<VTQR_ACCHoldPdovrdInc_flg>"
  [BINP_CAN3_outputs] -> Bus Selector34/1
  [VVMC_CalMeterSpeed_kph] -> ACC_Function/20(VVMC_CalMeterSpeed_kph)
  Bus Selector33/2 -> ACC_Function/26(VTQR_RrTMTqReq_Nm)  "<VTQR_RrTMTqReq_Nm>"
  [BDHP_outputs] -> Bus Selector4/1
  [VVMC_ACCReqSpdMemory_kph] -> ACC_Function/30(VVMC_ACCReqSpdMemory_kph)
  Bus Selector4/1 -> ACC_Function/32(VDHP_ActAPSPosn_pct)  "<VDHP_ActAPSPosn_pct>"
  Bus Selector2/1 -> ACC_Function/2(VTQD_DriverWhlTqDem_Nm)  "<VTQD_DriverWhlTqDem_Nm>"
  ACC_Function/1(VVMC_ACCCtrlAvail_flg) -> [VVMC_ACCCtrlAvail_flg]
  Bus Selector/1 -> ACC_Function/7(VINP_ACCRequireAccel_mps2)  "<VINP_ACCRequiredAccel_mps2>"
  [VVMC_ACCSpdCtrl_flg] -> ACC_Function/31(VVMC_ACCSpdCtrl_flg)
  [VVMC_LongAccP2_Gps] -> ACC_Function/15(VVMC_LongAcc_Gps)
  [BTQD_outputs] -> Bus Selector2/1
  Bus Selector/6 -> ACC_Function/12(VINP_MCPressure_bar)  "<VINP_MCPressure_bar>"
  [BINP_CAN1_outputs] -> Bus Selector/1
  [BINP_CAN2_outputs] -> Bus Selector35/1
  ACC_Function/5(VVMC_ADASNegReq_flg) -> [VVMC_ADASNegReq_flg]
  ACC_Function/3(VVMC_ADASWhlTqReq_Nm) -> [VVMC_ADASWhlTqReq_Nm]
  Bus Selector2/2 -> ACC_Function/3(VTQD_ExternalTqAllow_flg)  "<VTQD_ExternalTqAllow_flg>"
  [VVMC_TotalAvailBrkRgnTq_Nm] -> ACC_Function/22(VVMC_TotalAvailBrkRgnTq_Nm)
  [VVMC_EstSlope_Deg] -> ACC_Function/21(VVMC_EstSlope_Deg)
  ACC_Function/4(VVMC_ADASActive_flg) -> [VVMC_ADASActive_flg]
  [BINP_CAN4_outputs] -> Bus Selector14/1
  [BTQR_outputs] -> Bus Selector33/1
  [VVMC_TimeGapJudge_flag] -> ACC_Function/24(VVMC_TimeGapJudge_flag)
  Bus Selector/4 -> ACC_Function/10(VINP_ACCSetSpeed_enum)  "<VINP_ACCSetSpeed_enum>"
  Bus Selector2/3 -> ACC_Function/4(VTQD_LowIdleAccPedal_flg)  "<VTQD_LowIdleAccPedal_flg>"
  Bus Selector14/1 -> ACC_Function/18(VINP_RegenMode_enum)  "<VINP_RegenMode_enum>"
  [VVMC_AfterCtrlACCReqAccel_mps2] -> ACC_Function/29(VVMC_AfterCtrlACCReqAccel_mps2)
  Bus Selector/7 -> ACC_Function/13(VINP_ESCADASSta_enum)  "<VINP_ESCADASSta_enum>"
  Bus Selector/3 -> ACC_Function/9(VINP_VehSpeed_kph)  "<VINP_VehSpeed_kph>"
  Bus Selector34/2 -> ACC_Function/17(VINP_RrTMSpd_rpm)  "<VINP_RrTMSpd_rpm>"
  [VVMC_AccelTurnHold_flg] -> ACC_Function/23(VVMC_AccelTurnHold_flg)
  ACC_Function/2(VVMC_ACCPedalOvrd_flg) -> [VVMC_ACCPedalOvrd_flg]
  Bus Selector33/1 -> ACC_Function/25(VTQR_FrTMTqReq_Nm)  "<VTQR_FrTMTqReq_Nm>"
  Bus Selector2/4 -> ACC_Function/5(VTQD_ExtDoorAllow_flg)  "<VTQD_ExtDoorAllow_flg>"
  Bus Selector/8 -> ACC_Function/14(VINP_TargetType_enum)  "<VINP_TargetType_enum>"
  [task_time_s] -> ACC_Function/1(task_time_s)  "task_time_s"
  Bus Selector35/1 -> ACC_Function/28(VVMC_MeterIndSpeedForCalcu_kph)  "<VINP_METERKPHCalcu_kph>"
  Bus Selector/5 -> ACC_Function/11(VINP_ACCVehHoldReq_flg)  "<VINP_ACCVehHoldReq_flg>"
  [BINP_CAN1_outputs] -> Bus Selector37/1
  Bus Selector37/1 -> APS function/17(VINP_ADASACCSta_enum)  "<VINP_ADASACCSta_enum>"
  Bus Selector37/2 -> APS function/18(VINP_MCPressure_bar)  "<VINP_MCPressure_bar>"
  Bus Selector37/3 -> APS function/19(VINP_BrkSwSta_flg)  "<VINP_BrkSwSta_flg>"
  Bus Selector37/4 -> APS function/20(VINP_BrkPedalPos_pct)  "<VINP_BrkPedalPos_pct>"
  [VVMC_AllowSetSpd_flg] -> APS function/21(VVMC_AllowSetSpd_flg)
  [VVMC_LongAccelCalcuByVehSpd_gps] -> Long Acceleration Calculation/18(VVMC_LongAccelCalcuByVehSpd_gps)
  [VVMC_EstSlopeCal_Deg] -> Long Acceleration Calculation/19(VVMC_EstSlopeCal_Deg)
  Long Acceleration Calculation/8(VVMC_LongAccP2_Gps) -> [VVMC_LongAccP2_Gps]
  MSA function/5(VVMC_ExtraMSACtrlSta_enum) -> [VVMC_ExtraMSACtrlSta_enum]
  [VVMC_ExtraMSACtrlSta_enum] -> Bus Creator/54

== system vmc/VMC/ACC_Function ==
  task_time_s : Inport
  VTQD_DriverWhlTqDem_Nm : Inport  Port=2
  VTQD_ExternalTqAllow_flg : Inport  Port=3
  VTQD_LowIdleAccPedal_flg : Inport  Port=4
  VTQD_ExtDoorAllow_flg : Inport  Port=5
  VTQD_CreepBaseTqD_Nm : Inport  Port=6
  VINP_ACCRequireAccel_mps2 : Inport  Port=7
  VINP_ADASACCSta_enum : Inport  Port=8
  VINP_VehSpeed_kph : Inport  Port=9
  VINP_ACCSetSpeed_enum : Inport  Port=10
  VINP_ACCVehHoldReq_flg : Inport  Port=11
  VINP_MCPressure_bar : Inport  Port=12
  VINP_ESCADASSta_enum : Inport  Port=13
  VINP_TargetType_enum : Inport  Port=14
  VVMC_LongAcc_Gps : Inport  Port=15
  VINP_FrTMSpd_rpm : Inport  Port=16
  VINP_RrTMSpd_rpm : Inport  Port=17
  VINP_RegenMode_enum : Inport  Port=18
  VINP_SWCResUpSta_flg : Inport  Port=19
  VVMC_CalMeterSpeed_kph : Inport  Port=20
  VVMC_EstSlope_Deg : Inport  Port=21
  VVMC_TotalAvailBrkRgnTq_Nm : Inport  Port=22
  VVMC_AccelTurnHold_flg : Inport  Port=23
  VVMC_TimeGapJudge_flag : Inport  Port=24
  VTQR_FrTMTqReq_Nm : Inport  Port=25
  VTQR_RrTMTqReq_Nm : Inport  Port=26
  VTQR_ACCHoldPdovrdInc_flg : Inport  Port=27
  VVMC_MeterIndSpeedForCalcu_kph : Inport  Port=28
  VVMC_AfterCtrlACCReqAccel_mps2 : Inport  Port=29
  VVMC_ACCReqSpdMemory_kph : Inport  Port=30
  VVMC_ACCSpdCtrl_flg : Inport  Port=31
  VDHP_ActAPSPosn_pct : Inport  Port=32
  ACC Control Allow Judgement : Subsystem
  ACC Delta Torque Map and Calculation : Subsystem
  ACC Torque Source Determination : Subsystem
  Hand Shaking : Subsystem
  VVMC_ACCCtrlAvail_flg : Outport
  VVMC_ACCPedalOvrd_flg : Outport  Port=2
  VVMC_ADASWhlTqReq_Nm : Outport  Port=3
  VVMC_ADASActive_flg : Outport  Port=4
  VVMC_ADASNegReq_flg : Outport  Port=5
  wires:
  [VVMC_ACCPedalOvrd_flg] -> VVMC_ACCPedalOvrd_flg/1
  Hand Shaking/1(VVMC_ACCCtrlAvail_flg) -> [VVMC_ACCCtrlAvail_flg]
  VVMC_LongAcc_Gps/1 -> [VVMC_LongAcc_Gps]
  VINP_ADASACCSta_enum/1 -> [VINP_ADASACCSta_enum]
  VINP_ACCRequireAccel_mps2/1 -> [VINP_ACCRequireAccel_mps2]
  [VVMC_ACCCtrlAvail_flg] -> VVMC_ACCCtrlAvail_flg/1
  VTQD_ExternalTqAllow_flg/1 -> [VTQD_ExternalTqAllow_flg]
  VINP_VehSpeed_kph/1 -> [VINP_VehSpeed_kph]
  VTQD_DriverWhlTqDem_Nm/1 -> [VTQD_DriverWhlTqDem_Nm]
  [VVMC_LongAcc_Gps] -> ACC Delta Torque Map and Calculation/1(VVMC_LongAcc_Gps)
  [VINP_ACCRequireAccel_mps2] -> ACC Delta Torque Map and Calculation/2(VINP_ACCRequireAccel_mps2)
  [VINP_VehSpeed_kph] -> ACC Delta Torque Map and Calculation/3(VINP_VehSpeed_kph)
  [VTQD_DriverWhlTqDem_Nm] -> ACC Delta Torque Map and Calculation/4(VTQD_DriverWhlTqDem_Nm)
  ACC Delta Torque Map and Calculation/1(VVMC_ADASWhlTqCal_Nm) -> [VVMC_ADASWhlTqCal_Nm]
  [VTQD_DriverWhlTqDem_Nm] -> ACC Torque Source Determination/1(VTQD_DriverWhlTqDem_Nm)
  [VVMC_ADASWhlTqCal_Nm] -> ACC Torque Source Determination/2(VVMC_ADASWhlTqCal_Nm)
  ACC Torque Source Determination/1(VVMC_ACCPedalOvrd_flg) -> [VVMC_ACCPedalOvrd_flg]
  [VINP_ADASACCSta_enum] -> Hand Shaking/1(VINP_ADASACCSta_enum)
  Hand Shaking/2(VVMC_ADASActive_flg) -> [VVMC_ADASActive_flg]
  [VVMC_ADASActive_flg] -> ACC Delta Torque Map and Calculation/5(VVMC_ADASActive_flg)
  task_time_s/1 -> [task_time_s]
  [task_time_s] -> ACC Control Allow Judgement/1(task_time_s)
  [VTQD_ExternalTqAllow_flg] -> ACC Control Allow Judgement/2(VTQD_ExternalTqAllow_flag)
  ACC Control Allow Judgement/1(VVMC_ACCCtrlAllow_flg) -> [VVMC_ACCCtrlAllow_flg]
  [VVMC_ACCCtrlAllow_flg] -> Hand Shaking/2(VVMC_ACCCtrlAllow_flg)
  [VVMC_ADASActive_flg] -> VVMC_ADASActive_flg/1
  ACC Torque Source Determination/2(VVMC_ADASWhlTqReq_Nm) -> [VVMC_ADASWhlTqReq_Nm]
  [VVMC_ADASWhlTqReq_Nm] -> VVMC_ADASWhlTqReq_Nm/1
  [VVMC_ACCPedalOvrd_flg] -> ACC Delta Torque Map and Calculation/6(VVMC_ACCPedalOvrd_flg)
  [VINP_ADASACCSta_enum] -> ACC Torque Source Determination/3(VINP_ADASACCSta_enum)
  VTQD_LowIdleAccPedal_flg/1 -> [VTQD_LowIdleAccPedal_flg]
  [VTQD_LowIdleAccPedal_flg] -> ACC Torque Source Determination/4(VTQD_LowIdleAccPedal_flg)
  VINP_ACCSetSpeed_enum/1 -> [VINP_ACCSetSpeed_enum]
  [VINP_ACCSetSpeed_enum] -> ACC Delta Torque Map and Calculation/7(VINP_ACCSetSpeed_enum)
  VINP_ACCVehHoldReq_flg/1 -> [VINP_ACCVehHoldReq_flg]
  [VINP_ACCVehHoldReq_flg] -> ACC Delta Torque Map and Calculation/8(VINP_ACCVehHoldReq_flg)
  VINP_ESCADASSta_enum/1 -> [VINP_ESCADASSta_enum]
  VINP_RrTMSpd_rpm/1 -> [VINP_RrTMSpd_rpm]
  VINP_RegenMode_enum/1 -> [VINP_RegenMode_enum]
  VINP_MCPressure_bar/1 -> [VINP_MCPressure_bar]
  VINP_FrTMSpd_rpm/1 -> [VINP_FrTMSpd_rpm]
  [VVMC_ADASActive_flg] -> ACC Torque Source Determination/5(VVMC_ADASActive_flg)
  [VINP_RegenMode_enum] -> ACC Torque Source Determination/6(VINP_RegenMode_enum)
  [VINP_MCPressure_bar] -> ACC Delta Torque Map and Calculation/11(VINP_MCPressure_bar)
  [VINP_ESCADASSta_enum] -> ACC Delta Torque Map and Calculation/12(VINP_ESCADASSta_enum)
  [VINP_RrTMSpd_rpm] -> ACC Delta Torque Map and Calculation/10(VINP_RrTMSpd_rpm)
  [VINP_FrTMSpd_rpm] -> ACC Delta Torque Map and Calculation/9(VINP_FrTMSpd_rpm)
  [VINP_SWCResUpSta_flg] -> ACC Delta Torque Map and Calculation/15(VINP_SWCResUpSta_flg)
  [VVMC_CalMeterSpeed_kph] -> ACC Delta Torque Map and Calculation/14(VVMC_CalMeterSpeed_kph)
  [VINP_TargetType_enum] -> ACC Delta Torque Map and Calculation/13(VINP_TargetType_enum)
  VVMC_CalMeterSpeed_kph/1 -> [VVMC_CalMeterSpeed_kph]
  VINP_SWCResUpSta_flg/1 -> [VINP_SWCResUpSta_flg]
  VINP_TargetType_enum/1 -> [VINP_TargetType_enum]
  ACC Delta Torque Map and Calculation/2(VVMC_ADASNegReq_flg) -> [VVMC_ADASNegReq_flg]
  [VVMC_ADASNegReq_flg] -> VVMC_ADASNegReq_flg/1
  VVMC_EstSlope_Deg/1 -> [VVMC_EstSlope_Deg]
  [VVMC_EstSlope_Deg] -> ACC Delta Torque Map and Calculation/16(VVMC_EstSlope_Deg)
  [task_time_s] -> ACC Torque Source Determination/7(task_time_s)
  [VTQD_ExtDoorAllow_flg] -> ACC Control Allow Judgement/3(VTQD_ExtDoorAllow_flg)
  VTQD_ExtDoorAllow_flg/1 -> [VTQD_ExtDoorAllow_flg]
  VVMC_TotalAvailBrkRgnTq_Nm/1 -> ACC Delta Torque Map and Calculation/17(VVMC_TotalAvailBrkRgnTq_Nm)
  VVMC_AccelTurnHold_flg/1 -> ACC Delta Torque Map and Calculation/18(VVMC_AccelTurnHold_flg)
  [task_time_s] -> ACC Delta Torque Map and Calculation/19(task_time_s)
  VVMC_TimeGapJudge_flag/1 -> ACC Delta Torque Map and Calculation/20(VVMC_TimeGapJudge_flag)
  VTQR_FrTMTqReq_Nm/1 -> ACC Delta Torque Map and Calculation/21(VTQR_FrTMTqReq_Nm)
  VTQR_RrTMTqReq_Nm/1 -> ACC Delta Torque Map and Calculation/22(VTQR_RrTMTqReq_Nm)
  VVMC_MeterIndSpeedForCalcu_kph/1 -> ACC Delta Torque Map and Calculation/23(VVMC_MeterIndSpeedForCalcu_kph)
  [VINP_ADASACCSta_enum] -> ACC Delta Torque Map and Calculation/24(VINP_ADASACCSta_enum)
  VVMC_AfterCtrlACCReqAccel_mps2/1 -> ACC Delta Torque Map and Calculation/25(VVMC_AfterCtrlACCReqAccel_mps2)
  VVMC_ACCReqSpdMemory_kph/1 -> ACC Delta Torque Map and Calculation/26(VVMC_ACCReqSpdMemory_kph)
  VVMC_ACCSpdCtrl_flg/1 -> ACC Delta Torque Map and Calculation/27(VVMC_ACCSpdCtrl_flg)
  [VTQD_CreepBaseTqD_Nm] -> ACC Torque Source Determination/10(VTQD_CreepBaseTqD_Nm)
  [VINP_ACCVehHoldReq_flg] -> ACC Torque Source Determination/9(VINP_ACCVehHoldReq_flg)
  [VDHP_ActAPSPosn_pct] -> ACC Torque Source Determination/8(VDHP_ActAPSPosn_pct)
  VDHP_ActAPSPosn_pct/1 -> [VDHP_ActAPSPosn_pct]
  VTQD_CreepBaseTqD_Nm/1 -> [VTQD_CreepBaseTqD_Nm]
  VTQR_ACCHoldPdovrdInc_flg/1 -> ACC Torque Source Determination/11(VTQR_ACCHoldPdovrdInc_flg)

== system vmc/VMC/ACC_ReqAccelControl ==
  note: ACC Constant Speed Control Judgement
  note: ACC Constant Speed Control
  VINP_VehSpeed_kph : Inport
  VINP_ACCRequiredAccel_mps2 : Inport  Port=2
  VINP_ADASACCSta_enum : Inport  Port=3
  VVMC_MeterIndSpeedForCalcu_kph : Inport  Port=4
  AND3 : Logic  Inputs=3  AllPortsSameDT=off  OutDataTypeStr=boolean
  AND4 : Logic  AllPortsSameDT=off  OutDataTypeStr=boolean
  Add8 : Sum
  Add9 : Sum  Inputs=+-
  Constant57 : Constant  Value=KVMC_SpdCtrlEnBand_kph
  Constant58 : Constant  Value=KVMC_Veh2MeterSpdFactor_enum
  Constant59 : Constant  Value=KVMC_Veh2MeterSpdOffset_enum
  Constant60 : Constant  Value=KVMC_SpdCtrlDisBand_kph
  Constant62 : Constant  Value=MINUSONE_FLOAT
  Constant63 : Constant  Value=KVMC_SpdCtrlReqAccel_mps2
  Constant{64,66..68,90..92} (7 alike) : Constant  Value=ZERO_FLOAT
  Constant65 : Constant  Value=KVMC_Veh2MeterSpdLoFactor_enum
  Constant69 : Constant  Value=TRUE
  Constant70 : Constant  Value=FALSE
  Constant71 : Constant  Value=KVMC_ACCSpdCtrlSW_flg
  Constant86 : Constant  Value=ENUM_ADASACCSTA_ACTIVE
  Constant99 : Constant  Value=ENUM_ADASACCSTA_ACTIVE
  ConstantSpeedControl1 : Stateflow chart  TreatAsAtomicUnit=on
      settings: PortSchema="{\"entries\":[{\"content\":{\"sides\":[{\"content\":{\"connectorIds\":[\"In2\",\"In3\",\"In4\",\"In5\",\"In6\",\"In1\"]},\"type\":\"ConnectorPlacement.EquallySpacedRectSide\",\"uuid\":\"931d4d55-b643-4b97-a7aa-1deb2b509e83\"},{\"content\":{\"connectorIds\":[\"Out1\"],\"side\":\"RIGHT\"},\"type\":\"ConnectorPlacement.EquallySpacedRectSide\",\"uuid\":\"f2f28b13-6937-4f35-b44e-683edec0d4ba\"},{\"content\":{\"connectorIds\":[],\"side\":\"TOP\"},\"type\":\"ConnectorPlacement.EquallySpacedRectSide\",\"uuid\":\"e2886b86-de2a-4a68-b05f-bfb0f2051baf\"}]},\"type\":\"ConnectorPlacement.EquallySpacedConnector\",\"uuid\":\"cece4c76-e980-42e8-adab-da09fec387c1\"}],\"packageUris\":[\"http://schema.mathworks.com/mf0/Connector/R2020b\"],\"version\":\"1.0\"}"
  Divide11 : Product  Inputs=**
  Divide12 : Product  Inputs=**
  Merge2 : Merge
  NOT4 : Logic  Operator=NOT  AllPortsSameDT=off  OutDataTypeStr=boolean
  NOT5 : Logic  Operator=NOT  AllPortsSameDT=off  OutDataTypeStr=boolean
  OR4 : Logic  Operator=OR  AllPortsSameDT=off  OutDataTypeStr=boolean
  OR5 : Logic  AllPortsSameDT=off  OutDataTypeStr=boolean
  OR6 : Logic  Operator=OR  Inputs=3  AllPortsSameDT=off  OutDataTypeStr=boolean
  Relational Operator24 : RelationalOperator  Operator=<  OutDataTypeStr=boolean  RndMeth=Simplest
  Relational Operator25 : RelationalOperator  Operator=<  OutDataTypeStr=boolean  RndMeth=Simplest
  Relational Operator26 : RelationalOperator  Operator=>  OutDataTypeStr=boolean  RndMeth=Simplest
  Relational Operator33 : RelationalOperator  Operator===  OutDataTypeStr=boolean  RndMeth=Simplest
  Relational Operator34 : RelationalOperator  Operator=>  OutDataTypeStr=boolean  RndMeth=Simplest
  Relational Operator35 : RelationalOperator  Operator=<  OutDataTypeStr=boolean  RndMeth=Simplest
  Relational Operator36 : RelationalOperator  Operator=>  OutDataTypeStr=boolean  RndMeth=Simplest
  Relational Operator38 : RelationalOperator  Operator=~=  OutDataTypeStr=boolean  RndMeth=Simplest
  Round4 : Rounding  Operator=round
  Switch1 : Switch  Criteria=u2 > Threshold  Threshold=KVMC_Veh2MeterSpdLoBdy_kph
  Switch5 : Switch  Criteria=u2 > Threshold
  Triggered Subsystem4 : Subsystem  TreatAsAtomicUnit=on
  Triggered Subsystem5 : Subsystem  TreatAsAtomicUnit=on
  Unit Delay2 : UnitDelay  SampleTime=-1  HasFrameUpgradeWarning=on
  Unit Delay5 : UnitDelay  SampleTime=-1  HasFrameUpgradeWarning=on
  VVMC_AfterCtrlACCReqAccel_mps2 : Outport
  VVMC_ACCReqSpdMemory_kph : Outport  Port=2
  VVMC_ACCSpdCtrl_flg : Outport  Port=3
  wires:
  Add9/1 -> ConstantSpeedControl1/1(DeltaSpeed)
  Unit Delay5/1 -> Relational Operator34/1
  Relational Operator38/1 -> OR6/2
  [VVMC_MeterIndSpeedForCalcu_kph] -> Triggered Subsystem4/1(In1)
  Constant92/1 -> Relational Operator36/2
  Relational Operator25/1 -> OR6/1
  Constant59/1 -> Add8/1
  Triggered Subsystem4/2(Out2) -> Merge2/1
  [VINP_ACCRequiredAccel_mps2] -> Relational Operator36/1, Relational Operator26/1, Relational Operator25/1, Relational Operator35/1, Unit Delay5/1, Unit Delay2/1
  Merge2/1 -> [VVMC_ACCSpdCtrl_flg]  "VVMC_ACCSpdCtrl_flg"
  Constant67/1 -> Relational Operator25/2
  Constant71/1 -> AND4/2
  [VVMC_ACCSpdCtrl_flg] -> AND4/1
  Triggered Subsystem5/1(Out1) -> Merge2/2
  Add8/1 -> Switch1/1
  Switch1/1 -> Add9/1
  Relational Operator24/1 -> OR4/1
  Constant62/1 -> ConstantSpeedControl1/4(MINUSONE_FLOAT)
  Divide12/1 -> Switch1/3
  Unit Delay2/1 -> Relational Operator24/1
  OR5/1 -> AND3/3
  Constant64/1 -> ConstantSpeedControl1/6(ZERO_FLOAT)
  Divide11/1 -> Add8/2
  Constant70/1 -> Triggered Subsystem5/1(In1)
  Constant58/1 -> Divide11/1
  Constant60/1 -> ConstantSpeedControl1/3(KVMC_SpdCtrlDisBand_kph)
  OR6/1 -> Triggered Subsystem5/Trigger
  [VVMC_ACCReqSpdMemory_kph] -> Round4/1
  Constant99/1 -> Relational Operator38/2
  [VINP_ADASACCSta_enum] -> Relational Operator38/1
  Constant91/1 -> Relational Operator35/2
  [VINP_ADASACCSta_enum] -> Relational Operator33/1
  Constant86/1 -> Relational Operator33/2
  Relational Operator26/1 -> OR6/3
  Constant68/1 -> Relational Operator26/2
  AND4/1 -> Switch5/2
  Round4/1 -> Add9/2
  Relational Operator36/1 -> NOT4/1
  Constant90/1 -> Relational Operator34/2
  NOT5/1 -> OR5/1
  Switch5/1 -> [VVMC_AfterCtrlACCReqAccel_mps2]  "VVMC_AfterCtrlACCReqAccel_mps2"
  NOT4/1 -> OR5/2
  Constant66/1 -> Relational Operator24/2
  [VINP_VehSpeed_kph] -> Switch1/2, Divide12/1, Divide11/2
  ConstantSpeedControl1/1(ReqAccel) -> Switch5/1
  Relational Operator34/1 -> OR4/2
  Relational Operator33/1 -> AND3/2
  [VINP_ACCRequiredAccel_mps2] -> Switch5/3
  Constant65/1 -> Divide12/2
  Constant63/1 -> ConstantSpeedControl1/5(KVMC_SpdCtrlReqAccel_mps2)
  OR4/1 -> AND3/1
  Constant57/1 -> ConstantSpeedControl1/2(KVMC_SpdCtrlEnBand_kph)
  Relational Operator35/1 -> NOT5/1
  Constant69/1 -> Triggered Subsystem4/2(In2)
  Triggered Subsystem4/1(Out1) -> [VVMC_ACCReqSpdMemory_kph]  "VVMC_ACCReqSpdMemory_kph"
  AND3/1 -> Triggered Subsystem4/Trigger
  VINP_ACCRequiredAccel_mps2/1 -> [VINP_ACCRequiredAccel_mps2]
  VINP_ADASACCSta_enum/1 -> [VINP_ADASACCSta_enum]
  VVMC_MeterIndSpeedForCalcu_kph/1 -> [VVMC_MeterIndSpeedForCalcu_kph]
  VINP_VehSpeed_kph/1 -> [VINP_VehSpeed_kph]
  [VVMC_AfterCtrlACCReqAccel_mps2] -> VVMC_AfterCtrlACCReqAccel_mps2/1
  [VVMC_ACCReqSpdMemory_kph] -> VVMC_ACCReqSpdMemory_kph/1
  [VVMC_ACCSpdCtrl_flg] -> VVMC_ACCSpdCtrl_flg/1
